simulink model "SdC_lineare_progetto"  (R2023b)
settings: Solver=VariableStepAuto  StartTime=0.0  StopTime=0.01  RelTol=1e-3
libraries: cstblocks x2, simulink x2
settings Model: Creator=guidocarnevale  LastModifiedBy=leona

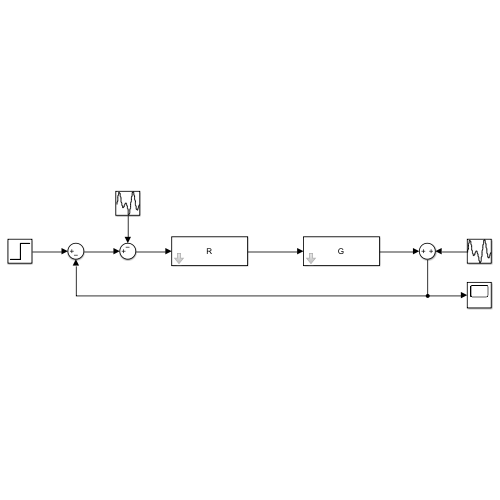
[thumbnail: Simulink's stored preview of the top-level diagram]
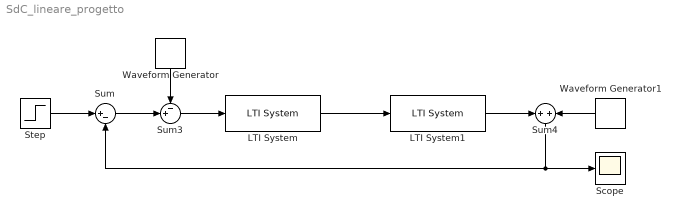
== system SdC_lineare_progetto ==
  LTI System : cstblocks/LTI System  Tag=R  sys=R  IC=[]  PadeOrder=0
  LTI System1 : cstblocks/LTI System  Tag=R  sys=G  IC=[]  PadeOrder=0
  Scope : Scope
  Step : Step  Time=0  SampleTime=0
  Sum : Sum  Inputs=|+-
  Sum3 : Sum  Inputs=-+|
  Sum4 : Sum  Inputs=+|+
  Waveform Generator : simulink/Sources/Waveform Generator  OutMin=[]  OutMax=[]  OutDataTypeStr=double  SelectedSignal=1  Signals=sin(1, 5e4, 0)+sin(1, 10e4, 0)+sin(1, 15e4, 0)+sin(1, 20e4, 0)  BlockNames=MultiportSwitch_3ff6c47c90af40d  SampleTime=0.000001
  Waveform Generator1 : simulink/Sources/Waveform Generator  OutMin=[]  OutMax=[]  OutDataTypeStr=double  SelectedSignal=1  Signals=sin(1, 0.1, 0)+sin(1, 0.2, 0)+sin(1, 0.3, 0)+sin(1, 0.4, 0)  BlockNames=MultiportSwitch_f54722ed020749d  SampleTime=0.01
  wires:
  Step/1 -> Sum/1
  LTI System/1 -> LTI System1/1
  LTI System1/1 -> Sum4/1
  Sum3/1 -> LTI System/1
  Waveform Generator1/1 -> Sum4/2
  Sum4/1 -> Scope/1, Sum/2
  Sum/1 -> Sum3/2
  Waveform Generator/1 -> Sum3/1
